simulink model "RoboController"  (Simulink 7.4)
settings: Solver=ode45  StartTime=0.0  StopTime=15  RelTol=1e-3
values from neighbouring files (symbols this model uses):
  Amp_to_Torque = 25.5/1000/GearRatio    (= 0.0765)    [parameter_setup.m]
  DampingRatio = 0.1*eye(4)    [parameter_setup.m]
  Force_Coupling_Mat = 1/Mass*[-sind(Thetas); cosd(Thetas); ones(size(Thetas))*1/alpha]    [parameter_setup.m]
  Friction_kinetic = U_kinetic * N_force    (= 19.62)    [parameter_setup.m]
  Friction_static = U_static*Mass* N_force    (= 117.72)    [parameter_setup.m]
  Max_Current = 2    [parameter_setup.m]
  Max_Voltage = 15    [parameter_setup.m]
  Motor_Ra = 1.2    [parameter_setup.m]
  MotorControllerType = Controller    (= 1)    [parameter_setup.m]
  MotorType = RealMotor    (= 0)    [parameter_setup.m]
  Slip_matrix = vel_coup_mat*pinv(vel_coup_mat)    [parameter_setup.m]
  Speed_to_Voltage = Speed_to_RPM/Volt_to_RPM    (= 3.0156943194)    [parameter_setup.m]
  vel_coup_mat = [-sind(Thetas'), cosd(Thetas'), ones(size(Thetas'))]    [parameter_setup.m]
  vel_scale_mat = vel_coup_mat*[1 0 0;0 1 0; 0 0 wheel_radius]    [parameter_setup.m]
  wheel_radius = 0.0254    [parameter_setup.m]
libraries: cstblocks x2, simulink x1
settings Model: Creator=Binaryblade  LastModifiedBy=Adrian Wong
settings DataIOCC: LimitDataPoints=off
settings OptimizationCC: InlineInvariantSignals=on  InitFltsAndDblsToZero=on
settings DebuggingCC: SaveWithParameterizedLinksMsg=none  SignalResolutionControl=TryResolveAllWithWarning  MultiTaskDSMMsg=warning  MultiTaskCondExecSysMsg=none  StrictBusMsg=None
settings RTWCC: SystemTargetFile=grt_malloc.tlc  TemplateMakefile=grt_malloc_default_tmf  Description=Generic Real-Time Target with dynamic memory allocation  ProcessScript=grt_malloc_make_rtw_hook  IncludeERTFirstTime=on  RTWCompilerOptimization=On
settings GRTTargetCC: UseMalloc=on  ExtModeMexFile=noextcomm

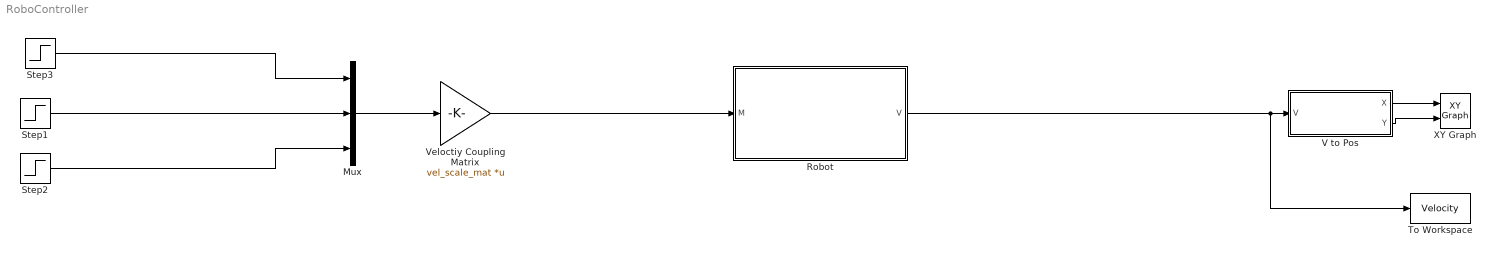
== system RoboController ==
  Mux : Mux  Inputs=3
  Robot : Subsystem
  Step1 : Step  Time=2.5  SampleTime=0
  Step2 : Step  Time=4  After=3  SampleTime=0
  Step3 : Step  SampleTime=0
  To Workspace : ToWorkspace  VariableName=Velocity  SampleTime=-1  SaveFormat=Array
  V to Pos : Subsystem
  Veloctiy Coupling Matrix : Gain  Gain=vel_scale_mat  Multiplication=Matrix(K*u)  ParameterDataType=sfix(16)  ParameterScaling=2^0  OutDataType=sfix(16)  OutScaling=2^0
  XY Graph : simulink/Sinks/XY Graph  SystemSampleTime=-1  xmin=-3.5  xmax=3.5  ymin=-2.5  ymax=2.5  st=-1
  wires:
  V to Pos/1(X) -> XY Graph/1
  V to Pos/2(Y) -> XY Graph/2
  Robot/1(V) -> To Workspace/1, V to Pos/1(V)
  Mux/1 -> Veloctiy Coupling Matrix/1
  Step3/1 -> Mux/1
  Step1/1 -> Mux/2
  Step2/1 -> Mux/3
  Veloctiy Coupling Matrix/1 -> Robot/1(M)

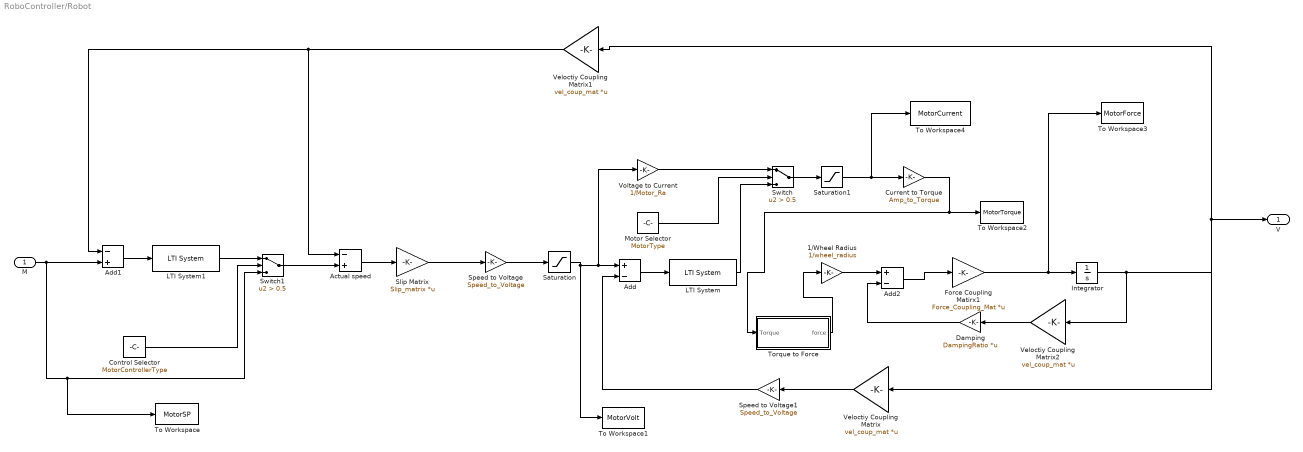
== system RoboController/Robot ==
  M : Inport  OutDataType=sfix(16)  OutScaling=2^0
  1/Wheel Radius : Gain  Gain=1/wheel_radius  ParameterDataType=sfix(16)  ParameterScaling=2^0  OutDataType=sfix(16)  OutScaling=2^0
  Actual speed : Sum  Inputs=-+  OutDataType=fixdt(1, 16)  OutScaling=2^-10
  Add : Sum  Inputs=+-  OutDataType=sfix(16)  OutScaling=2^-10
  Add1 : Sum  Inputs=-+  OutDataType=sfix(16)  OutScaling=2^-10
  Add2 : Sum  Inputs=+-  OutDataType=sfix(16)  OutScaling=2^-10
  Control Selector : Constant  Value=MotorControllerType  OutDataType=sfix(16)  OutScaling=2^0
  Current to Torque : Gain  Gain=Amp_to_Torque  ParameterDataType=sfix(16)  ParameterScaling=2^0  OutDataType=sfix(16)  OutScaling=2^0
  Damping : Gain  Gain=DampingRatio  Multiplication=Matrix(K*u)  ParameterDataType=sfix(16)  ParameterScaling=2^0  OutDataType=sfix(16)  OutScaling=2^0
  Force Coupling Matirx1 : Gain  Gain=Force_Coupling_Mat  Multiplication=Matrix(K*u)  ParameterDataType=sfix(16)  ParameterScaling=2^0  OutDataType=sfix(16)  OutScaling=2^0
  Integrator : Integrator
  LTI System : cstblocks/LTI System  SystemSampleTime=-1  sys=MotorTF  IC=[]
  LTI System1 : cstblocks/LTI System  SystemSampleTime=-1  sys=MotorController  IC=[]
  Motor Selector : Constant  Value=MotorType  OutDataType=sfix(16)  OutScaling=2^0
  Saturation : Saturate  UpperLimit=Max_Voltage  LowerLimit=-Max_Voltage
  Saturation1 : Saturate  UpperLimit=Max_Current  LowerLimit=-Max_Current
  Slip Matrix : Gain  Gain=Slip_matrix  Multiplication=Matrix(K*u)  ParameterDataType=sfix(16)  ParameterScaling=2^0  OutDataType=sfix(16)  OutScaling=2^0
  Speed to Voltage : Gain  Gain=Speed_to_Voltage  ParameterDataType=sfix(16)  ParameterScaling=2^0  OutDataType=sfix(16)  OutScaling=2^0
  Speed to Voltage1 : Gain  Gain=Speed_to_Voltage  ParameterDataType=sfix(16)  ParameterScaling=2^0  OutDataType=sfix(16)  OutScaling=2^0
  Switch : Switch  Criteria=u2 > Threshold  Threshold=0.5  OutDataType=sfix(16)  OutScaling=2^0
  Switch1 : Switch  Criteria=u2 > Threshold  Threshold=0.5  OutDataType=sfix(16)  OutScaling=2^0
  To Workspace : ToWorkspace  VariableName=MotorSP  SampleTime=-1  SaveFormat=Array
  To Workspace1 : ToWorkspace  VariableName=MotorVolt  SampleTime=-1  SaveFormat=Array
  To Workspace2 : ToWorkspace  VariableName=MotorTorque  SampleTime=-1  SaveFormat=Array
  To Workspace3 : ToWorkspace  VariableName=MotorForce  SampleTime=-1  SaveFormat=Array
  To Workspace4 : ToWorkspace  VariableName=MotorCurrent  SampleTime=-1  SaveFormat=Array
  Torque to Force : Subsystem
  Veloctiy Coupling Matrix : Gain  Gain=vel_coup_mat  Multiplication=Matrix(K*u)  ParameterDataType=sfix(16)  ParameterScaling=2^0  OutDataType=sfix(16)  OutScaling=2^0
  Veloctiy Coupling Matrix1 : Gain  Gain=vel_coup_mat  Multiplication=Matrix(K*u)  ParameterDataType=sfix(16)  ParameterScaling=2^0  OutDataType=sfix(16)  OutScaling=2^0
  Veloctiy Coupling Matrix2 : Gain  Gain=vel_coup_mat  Multiplication=Matrix(K*u)  ParameterDataType=sfix(16)  ParameterScaling=2^0  OutDataType=sfix(16)  OutScaling=2^0
  Voltage to Current : Gain  Gain=1/Motor_Ra  ParameterDataType=sfix(16)  ParameterScaling=2^0  OutDataType=sfix(16)  OutScaling=2^0
  V : Outport  OutDataType=sfix(16)  OutScaling=2^0
  wires:
  Current to Torque/1 -> To Workspace2/1, Torque to Force/1(Torque)
  Integrator/1 -> Veloctiy Coupling Matrix/1, V/1, Veloctiy Coupling Matrix1/1, Veloctiy Coupling Matrix2/1
  Veloctiy Coupling Matrix/1 -> Speed to Voltage1/1
  Add/1 -> LTI System/1
  Saturation/1 -> To Workspace1/1, Voltage to Current/1, Add/1
  Speed to Voltage1/1 -> Add/2
  M/1 -> Add1/2, To Workspace/1, Switch1/3
  Voltage to Current/1 -> Switch/1
  LTI System/1 -> Switch/3
  Switch/1 -> Saturation1/1
  Motor Selector/1 -> Switch/2
  Add1/1 -> LTI System1/1
  LTI System1/1 -> Switch1/1
  Control Selector/1 -> Switch1/2
  Speed to Voltage/1 -> Saturation/1
  Saturation1/1 -> Current to Torque/1, To Workspace4/1
  Force Coupling Matirx1/1 -> To Workspace3/1, Integrator/1
  1/Wheel Radius/1 -> Add2/1
  Add2/1 -> Force Coupling Matirx1/1
  Damping/1 -> Add2/2
  Veloctiy Coupling Matrix1/1 -> Add1/1, Actual speed/1
  Veloctiy Coupling Matrix2/1 -> Damping/1
  Switch1/1 -> Actual speed/2
  Actual speed/1 -> Slip Matrix/1
  Slip Matrix/1 -> Speed to Voltage/1
  Torque to Force/1(force) -> 1/Wheel Radius/1

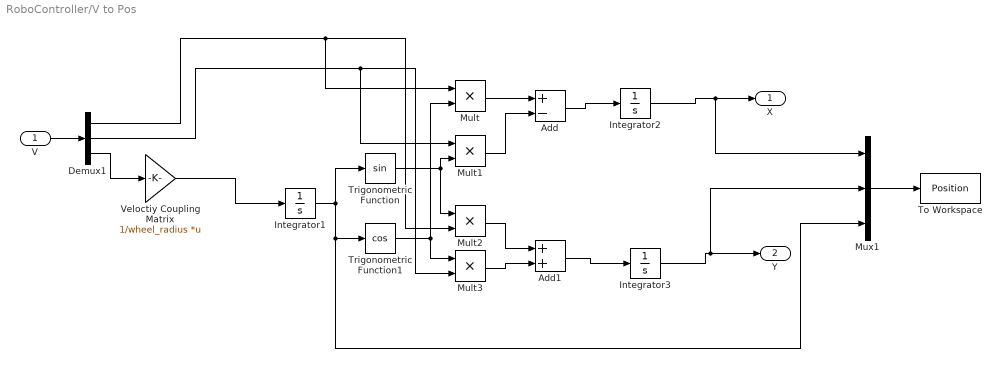
== system RoboController/V to Pos ==
  V : Inport  OutDataType=sfix(16)  OutScaling=2^0
  Add : Sum  Inputs=+-  OutDataType=sfix(16)  OutScaling=2^-10
  Add1 : Sum  OutDataType=sfix(16)  OutScaling=2^-10
  Demux1 : Demux  Outputs=3
  Integrator1 : Integrator
  Integrator2 : Integrator
  Integrator3 : Integrator
  Mult{,1..3} (4 alike) : Product  Inputs=**  OutDataType=sfix(16)  OutScaling=2^-10
  Mux1 : Mux  Inputs=3
  To Workspace : ToWorkspace  VariableName=Position  SampleTime=-1  SaveFormat=Array
  Trigonometric Function : Trigonometry
  Trigonometric Function1 : Trigonometry  Operator=cos
  Veloctiy Coupling Matrix : Gain  Gain=1/wheel_radius  Multiplication=Matrix(K*u)  ParameterDataType=sfix(16)  ParameterScaling=2^0  OutDataType=sfix(16)  OutScaling=2^0
  X : Outport  OutDataType=sfix(16)  OutScaling=2^0
  Y : Outport  Port=2  OutDataType=sfix(16)  OutScaling=2^0
  wires:
  Integrator1/1 -> Trigonometric Function/1, Trigonometric Function1/1, Mux1/3
  Trigonometric Function1/1 -> Mult/2, Mult3/1
  Mult/1 -> Add/1
  Mult1/1 -> Add/2
  Trigonometric Function/1 -> Mult1/2, Mult2/1
  Demux1/2 -> Mult1/1, Mult3/2
  Mult3/1 -> Add1/2
  Mult2/1 -> Add1/1
  Add/1 -> Integrator2/1
  Integrator2/1 -> X/1, Mux1/1
  Add1/1 -> Integrator3/1
  Integrator3/1 -> Y/1, Mux1/2
  Mux1/1 -> To Workspace/1
  Demux1/1 -> Mult/1, Mult2/2
  V/1 -> Demux1/1
  Demux1/3 -> Veloctiy Coupling Matrix/1
  Veloctiy Coupling Matrix/1 -> Integrator1/1

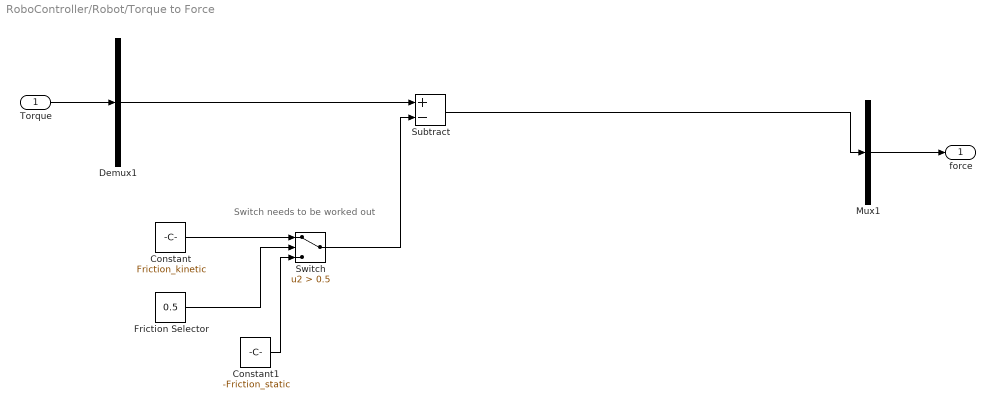
== system RoboController/Robot/Torque to Force ==
  note: Switch needs to be worked out
  Torque : Inport  OutDataType=sfix(16)  OutScaling=2^0
  Constant : Constant  Value=Friction_kinetic  OutDataType=fixdt(1, 16)  OutScaling=2^0
  Constant1 : Constant  Value=-Friction_static  OutDataType=fixdt(1, 16)  OutScaling=2^0
  Demux1 : Demux  Outputs=1
  Friction Selector : Constant  Value=0.5  OutDataType=sfix(16)  OutScaling=2^0
  Mux1 : Mux  Inputs=1
  Subtract : Sum  Inputs=+-  OutDataType=fixdt(1, 16)  OutScaling=2^-10
  Switch : Switch  Criteria=u2 > Threshold  Threshold=0.5  OutDataType=sfix(16)  OutScaling=2^0
  force : Outport  OutDataType=fixdt(1, 16)  OutScaling=2^0
  wires:
  Mux1/1 -> force/1
  Torque/1 -> Demux1/1
  Friction Selector/1 -> Switch/2
  Constant1/1 -> Switch/3
  Constant/1 -> Switch/1
  Switch/1 -> Subtract/2
  Demux1/1 -> Subtract/1
  Subtract/1 -> Mux1/1
